simulink model "Position_Generator"  (R2017a)
settings: Solver=ode2  StartTime=0.0  StopTime=inf  FixedStep=0.001  RelTol=1e-3  EnableMultiTasking=on
model workspace (MAT data in the model file):
  Sig = Simulink.Signal
  Sig.DataType = 'auto'
  Sig.Dimensions = -1
  Sig.DimensionsMode = 'auto'
  Sig.Complexity = 'auto'
  Sig.SampleTime = -1
  Sig.SamplingMode = 'auto'
  video_step_size = 0.06
libraries: quarc_library x8, simulink x1
settings Model: SimulationMode=external  Creator=Admin  LastModifiedBy=mbohra
settings SolverCC: PositivePriorityOrder=on
settings OptimizationCC: LifeSpan=inf
settings DebuggingCC: ParameterPrecisionLossMsg=none  SFUnexpectedBacktrackingDiag=warning  SFNoUnconditionalDefaultTransitionDiag=warning  SFExecutionAtInitializationDiag=none
settings HardwareCC: ProdBitPerLong=64  ProdLargestAtomicFloat=None  ProdHWDeviceType=Intel->x86-64
settings RTWCC: SystemTargetFile=quarc_linux_x64.tlc  TemplateMakefile=quarc_linux_x64_tmf  Description=QUARC Linux x64 Target
settings STFCustomTargetCC: TargetLibSuffix=.a  TargetPreCompLibLocation=C:\PROGRA~3\QUARC\lib\2017a\LINUX_~1\release  ConcurrentExecutionCompliant=on  SystemTargetFile=quarc_linux_x64.tlc
settings GRTTargetCC: TargetLibSuffix=.a  TargetPreCompLibLocation=C:\PROGRA~3\QUARC\lib\2017a\LINUX_~1\release  TargetLangStandard=C89/C90 (ANSI)  ParMdlRefBuildCompliant=off  CompOptLevelCompliant=off  CombineOutputUpdateFcns=off  MatFileLogging=off  CPPClassGenCompliant=off  GRTInterface=on  UseToolchainInfoCompliant=off  ExtMode=on  ExtModeMexFile=quarc_comm  ExtModeMexArgs='-w -d /tmp -uri %u -IP_address tcpip://192.168.2.3:18666','tcpip://qondor888864.local:17002?retries=10'
settings ConfigComp: CovMetricSettings=dw  CovHtmlReporting=on  CovSaveCumulativeToWorkspaceVar=on  CovSaveSingleToWorkspaceVar=on  CovExternalEMLEnable=off

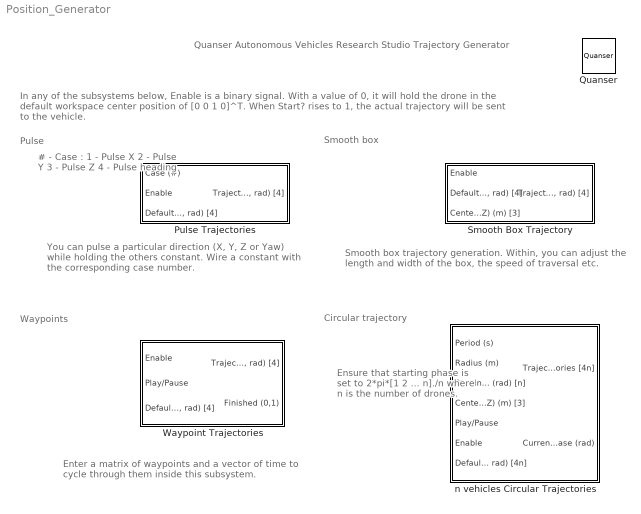
== system Position_Generator ==
  note: Ensure that starting phase is set to
      |  2*pi*[1 2 ... n]./n
      | where n is the number of drones.
  note: Circular trajectory
  note: Waypoints
  note: Smooth box
  note: Pulse
  note: You can pulse a particular direction (X, Y, Z or Yaw)
      | while holding the others constant. Wire a constant
      | with the corresponding case number.
  note: In any of the subsystems below, Enable is a binary signal. With a value of 0, it will hold the drone in the default workspace center position of [0 0 1 0]^T. When Start? rises to 1, the actual trajectory will be sent to the vehicle.
  note: # - Case :
      | 1 - Pulse X
      | 2 - Pulse Y
      | 3 - Pulse Z
      | 4 - Pulse heading
  note: Quanser Autonomous Vehicles Research Studio
      | Trajectory Generator
  note: Enter a matrix of waypoints and a vector of time
      | to cycle through them inside this subsystem.
  note: Smooth box trajectory generation. Within, you can adjust
      | the length and width of the box, the speed of traversal etc.
  Pulse Trajectories : Subsystem
  Quanser : quarc_library/Logos/Quanser
  Smooth Box Trajectory : Subsystem
  Waypoint Trajectories : Subsystem
  n vehicles Circular Trajectories : Subsystem

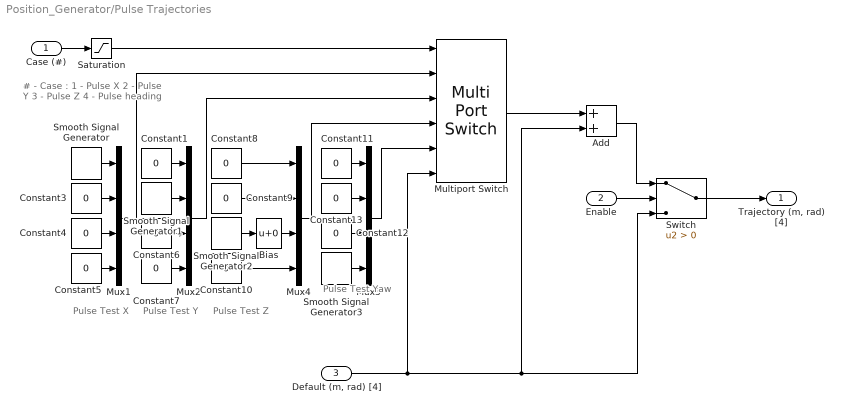
== system Position_Generator/Pulse Trajectories ==
  note: Pulse
      | Test Y
  note: Pulse
      | Test X
  note: Pulse
      | Test Z
  note: Pulse
      | Test
      | Yaw
  note: # - Case :
      | 1 - Pulse X
      | 2 - Pulse Y
      | 3 - Pulse Z
      | 4 - Pulse heading
  Case (#) : Inport
  Enable : Inport  Port=2
  "Default (m, rad) [4]" : Inport  Port=3
  Add : Sum
  Bias : Bias
  Constant{1,3..13} (12 alike) : Constant  Value=0
  Multiport Switch : MultiPortSwitch  Inputs=5
  Mux{1..2,4..5} (4 alike) : Mux  Inputs=[1 1 1 1]
  Saturation : Saturate  UpperLimit=5  LowerLimit=1
  Smooth Signal Generator : quarc_library/Sources/Signals/Smooth Signal Generator  signal_type=Square  source=Internal (dialog parameters)  amplitude=0.75  frequency=0.05  initial_phase=0  sample_time=qc_get_step_size  output_cos=off
      settings: SourceProductName=QUARC Targets
  Smooth Signal Generator1 : quarc_library/Sources/Signals/Smooth Signal Generator  signal_type=Square  source=Internal (dialog parameters)  amplitude=0.75  frequency=0.05  initial_phase=0  sample_time=qc_get_step_size  output_cos=off
      settings: SourceProductName=QUARC Targets
  Smooth Signal Generator2 : quarc_library/Sources/Signals/Smooth Signal Generator  signal_type=Square  source=Internal (dialog parameters)  amplitude=0.5  frequency=0.05  initial_phase=0  sample_time=qc_get_step_size  output_cos=off
      settings: SourceProductName=QUARC Targets
  Smooth Signal Generator3 : quarc_library/Sources/Signals/Smooth Signal Generator  signal_type=Square  source=Internal (dialog parameters)  amplitude=pi/4  frequency=0.05  initial_phase=0  sample_time=qc_get_step_size  output_cos=off
      settings: SourceProductName=QUARC Targets
  Switch : Switch  Criteria=u2 > Threshold
  "Trajectory (m, rad) [4]" : Outport
  wires:
  Constant3/1 -> Mux1/2
  Smooth Signal Generator/1 -> Mux1/1
  Constant5/1 -> Mux1/4
  Constant4/1 -> Mux1/3
  Mux1/1 -> Multiport Switch/2
  Case (#)/1 -> Saturation/1
  Mux2/1 -> Multiport Switch/3
  Constant6/1 -> Mux2/3
  Constant7/1 -> Mux2/4
  Constant1/1 -> Mux2/1
  Smooth Signal Generator1/1 -> Mux2/2
  Constant9/1 -> Mux4/2
  Constant8/1 -> Mux4/1
  Constant10/1 -> Mux4/4
  Smooth Signal Generator2/1 -> Bias/1
  Bias/1 -> Mux4/3
  Constant13/1 -> Mux5/2
  Constant11/1 -> Mux5/1
  Smooth Signal Generator3/1 -> Mux5/4
  Constant12/1 -> Mux5/3
  Mux4/1 -> Multiport Switch/4
  Mux5/1 -> Multiport Switch/5
  Saturation/1 -> Multiport Switch/1
  "Default (m, rad) [4]"/1 -> Add/2, Switch/3, Multiport Switch/6
  Switch/1 -> "Trajectory (m, rad) [4]"/1
  Enable/1 -> Switch/2
  Multiport Switch/1 -> Add/1
  Add/1 -> Switch/1

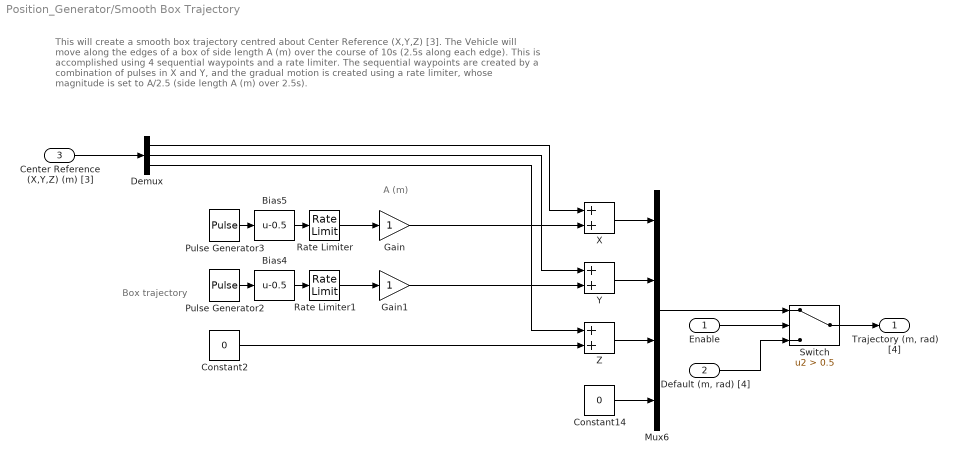
== system Position_Generator/Smooth Box Trajectory ==
  note: A (m)
  note: This will create a smooth box trajectory centred about Center Reference (X,Y,Z) [3]. The Vehicle will move along the edges of a box
      | of side length A (m) over the course of 10s (2.5s along each edge).
      |
      | This is accomplished using 4 sequential waypoints and a rate limiter. The sequential waypoints are created by a combination of
      | pulses in X and Y, and the gradual motion is created using a rate limiter, whose magnitude is set to A/2.5 (side length A (m) over 2.5s).
  note: Box
      | trajectory
  Enable : Inport
  "Default (m, rad) [4]" : Inport  Port=2
  Center Reference (X,Y,Z) (m) [3] : Inport  Port=3
  Bias4 : Bias  Bias=-0.5
  Bias5 : Bias  Bias=-0.5
  Constant14 : Constant  Value=0
  Constant2 : Constant  Value=0
  Demux : Demux  Outputs=3
  Gain : Gain
  Gain1 : Gain
  Mux6 : Mux  Inputs=[1 1 1 1]
  Pulse Generator2 : DiscretePulseGenerator  PulseType=Time based  Period=10  PulseWidth=50
  Pulse Generator3 : DiscretePulseGenerator  PulseType=Time based  Period=10  PulseWidth=50  PhaseDelay=-2.5
  Rate Limiter : RateLimiter  RisingSlewLimit=1/2.5  FallingSlewLimit=-1/2.5  SampleTimeMode=inherited  InitialCondition=0.5
  Rate Limiter1 : RateLimiter  RisingSlewLimit=1/2.5  FallingSlewLimit=-1/2.5  SampleTimeMode=inherited  InitialCondition=0.5
  Switch : Switch  Criteria=u2 > Threshold  Threshold=0.5
  X : Sum
  Y : Sum
  Z : Sum
  "Trajectory (m, rad) [4]" : Outport
  wires:
  Constant14/1 -> Mux6/4
  Bias5/1 -> Rate Limiter/1
  Pulse Generator3/1 -> Bias5/1
  Pulse Generator2/1 -> Bias4/1
  Bias4/1 -> Rate Limiter1/1
  Rate Limiter1/1 -> Gain1/1
  Rate Limiter/1 -> Gain/1
  "Default (m, rad) [4]"/1 -> Switch/3
  Switch/1 -> "Trajectory (m, rad) [4]"/1
  Enable/1 -> Switch/2
  Gain1/1 -> Y/2
  Demux/3 -> Z/1
  Center Reference (X,Y,Z) (m) [3]/1 -> Demux/1
  Demux/1 -> X/1
  Demux/2 -> Y/1
  Gain/1 -> X/2
  Constant2/1 -> Z/2
  X/1 -> Mux6/1
  Y/1 -> Mux6/2
  Z/1 -> Mux6/3
  Mux6/1 -> Switch/1

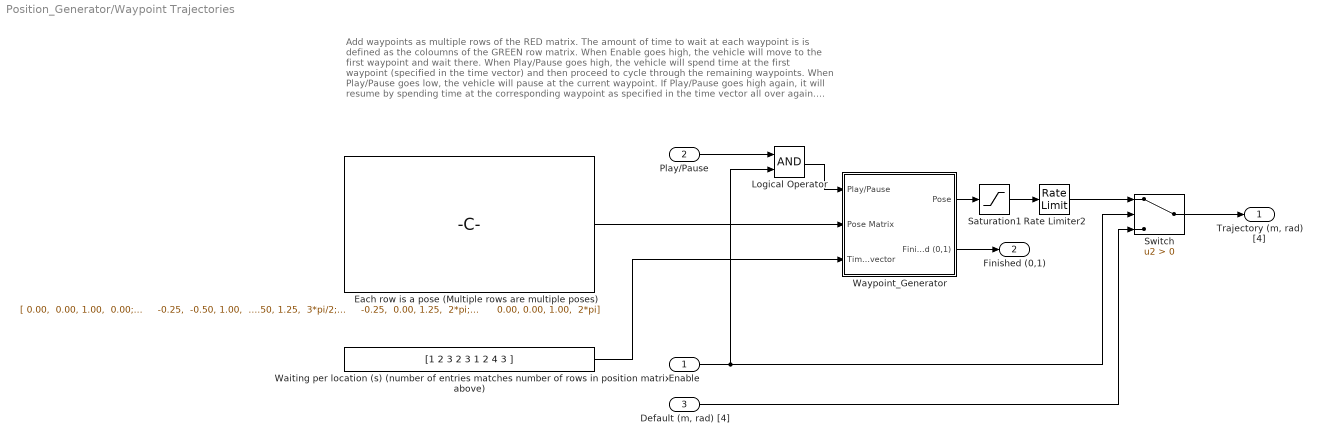
== system Position_Generator/Waypoint Trajectories ==
  note: Add waypoints as multiple rows of the RED matrix. The amount of time to wait at each waypoint is is defined as the coloumns of the GREEN row matrix.
      |
      | When Enable goes high, the vehicle will move to the first waypoint and wait there.
      | When Play/Pause goes high, the vehicle will spend time at the first waypoint (specified in the time vector) and then proceed to cycle through the remaining waypoints.
      | When Play/Pause goes low, the vehicle will pause at the current waypoint. If Play/Pause goes high again, it will resume by spending time at the corresponding waypoint
      | as specified in the time vector all over again.
      | When Enable goes low at any point, the vehicle will move back to the Default pose.
  Enable : Inport
  Play/Pause : Inport  Port=2
  "Default (m, rad) [4]" : Inport  Port=3
  Each row is a pose (Multiple rows are multiple poses) : Constant  Value=|
      | [ 0.00,  0.00, 1.00,  0.00;...
      |     -0.25,  -0.50, 1.00,  0.00;...
      |     -0.25, -0.50, 0.75,  0.00;...
      |      0.75, -0.50, 0.75,  pi/2;...
      |      0.75, -0.50, 1.25,  pi/2;...
      |      0.75,  0.50, 1.25,  pi;...
      |     -0.25,  0.50, 1.25,  3*pi/2;...
      |     -0.25,  0.00, 1.25,  2*pi;...
      |      0.00, 0.00, 1.00,  2*pi]
  Logical Operator : Logic  AllPortsSameDT=off  OutDataTypeStr=boolean
  Rate Limiter2 : RateLimiter  RisingSlewLimit=[1/3 1/3 1/6 pi/6]  FallingSlewLimit=[-1/3 -1/3 -1/6 -pi/6]  SampleTimeMode=inherited
  Saturation1 : Saturate  UpperLimit=[1.5 1.5 2 3*pi]  LowerLimit=[-1.5 -1.5 0 -3*pi]
  Switch : Switch  Criteria=u2 > Threshold
  Waiting per location (s) (number of entries matches number of rows in position matrix above) : Constant  Value=[1 2 3 2 3 1 2 4 3 ]
  Waypoint_Generator : Subsystem
  "Trajectory (m, rad) [4]" : Outport
  Finished (0,1) : Outport  Port=2
  wires:
  Waypoint_Generator/1(Pose) -> Saturation1/1
  Waiting per location (s) (number of entries matches number of rows in position matrix above)/1 -> Waypoint_Generator/3(Time vector)
  Each row is a pose (Multiple rows are multiple poses)/1 -> Waypoint_Generator/2(Pose Matrix)
  Saturation1/1 -> Rate Limiter2/1
  Play/Pause/1 -> Logical Operator/1
  Rate Limiter2/1 -> Switch/1
  Enable/1 -> Logical Operator/2, Switch/2
  "Default (m, rad) [4]"/1 -> Switch/3
  Switch/1 -> "Trajectory (m, rad) [4]"/1
  Logical Operator/1 -> Waypoint_Generator/1(Play/Pause)
  Waypoint_Generator/2(Finished (0,1)) -> Finished (0,1)/1

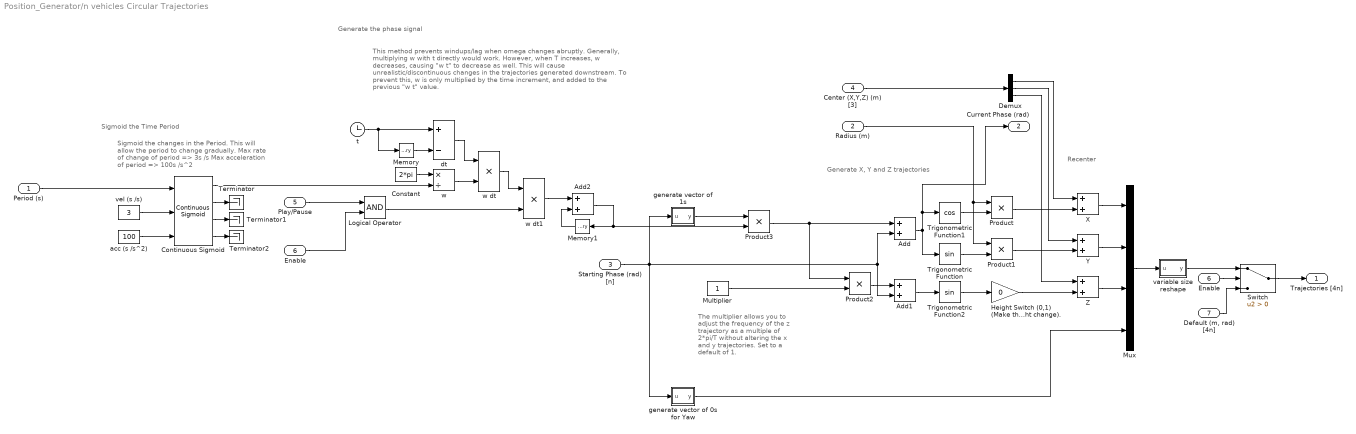
== system Position_Generator/n vehicles Circular Trajectories ==
  note: Recenter
  note: Generate X, Y and Z trajectories
  note: Generate the phase signal
  note: Sigmoid the changes in the Period. This will
      | allow the period to change gradually.
      | Max rate of change of period => 3s /s
      | Max acceleration of period => 100s /s^2
  note: Sigmoid the Time Period
  note: The multiplier allows you to adjust the frequency of the z trajectory as a multiple of 2*pi/T without altering the x and y trajectories. Set to a default of 1.
  note: This method prevents windups/lag when omega changes abruptly. Generally, multiplying w with t directly would work. However, when T increases, w decreases, causing "w t" to decrease as well. This will cause unrealistic/discontinuous changes in the trajectories generated downstream.
      |
      | To prevent this, w is only multiplied by the time increment, and added to the previous "w t" value.
  Period (s) : Inport
  Radius (m) : Inport  Port=2
  Starting Phase (rad) [n] : Inport  Port=3
  Center (X,Y,Z) (m) [3] : Inport  Port=4
  Play/Pause : Inport  Port=5
  Enable : Inport  Port=6
  "Default (m, rad) [4n]" : Inport  Port=7
  " Enable " : InportShadow  Port=6
  Add : Sum
  Add1 : Sum
  Add2 : Sum
  Constant : Constant  Value=2*pi
  Continuous Sigmoid : quarc_library/Sources/Sigmoids/Continuous Sigmoid  params_source=External (input ports)  max_velocity=2  max_acceleration=10  initial_position=10  initial_velocity=0  hold_off=0.5  input_sample_time=-1  output_sample_time=qc_get_step_size
      settings: SourceProductName=QUARC Targets
  Demux : Demux  Outputs=3
  Height Switch (0,1) (Make this 0 to disable height change). : Gain  Gain=0
  Logical Operator : Logic  AllPortsSameDT=off  OutDataTypeStr=boolean
  Memory : Memory
  Memory1 : Memory
  Multiplier : Constant
  Mux : Mux
  Product{,1..3} (4 alike) : Product
  Switch : Switch  Criteria=u2 > Threshold
  Terminator : Terminator
  Terminator1 : Terminator
  Terminator2 : Terminator
  Trigonometric Function : Trigonometry
  Trigonometric Function1 : Trigonometry  Operator=cos
  Trigonometric Function2 : Trigonometry
  X : Sum
  Y : Sum
  Z : Sum
  acc (s /s^2) : Constant  Value=100
  dt : Sum  Inputs=+-
  generate vector of 0s for Yaw : MATLAB Function  TreatAsAtomicUnit=on
  generate vector of 1s : MATLAB Function  TreatAsAtomicUnit=on
  t : Clock
  variable size reshape : MATLAB Function  TreatAsAtomicUnit=on
  vel (s /s) : Constant  Value=3
  w : Product  Inputs=*/
  w dt : Product
  w dt1 : Product
  Trajectories [4n] : Outport
  Current Phase (rad) : Outport  Port=2
  wires:
  Trigonometric Function/1 -> Product1/2
  Trigonometric Function1/1 -> Product/2
  Height Switch (0,1) (Make this 0 to disable height change)./1 -> Z/2
  Product1/1 -> Y/2
  Product/1 -> X/2
  Radius (m)/1 -> Product/1, Product1/1
  generate vector of 0s for Yaw/1(y) -> Mux/4
  Continuous Sigmoid/4 -> Terminator2/1
  Period (s)/1 -> Continuous Sigmoid/1
  Continuous Sigmoid/2 -> Terminator/1
  Continuous Sigmoid/3 -> Terminator1/1
  acc (s /s^2)/1 -> Continuous Sigmoid/3
  vel (s /s)/1 -> Continuous Sigmoid/2
  Add1/1 -> Trigonometric Function2/1
  Multiplier/1 -> Product2/2
  Product2/1 -> Add1/1
  Starting Phase (rad) [n]/1 -> Add/2, Add1/2, generate vector of 1s/1(u), generate vector of 0s for Yaw/1(u)
  Add2/1 -> Memory1/1, Product3/2
  Add/1 -> Current Phase (rad)/1, Trigonometric Function1/1, Trigonometric Function/1
  Center (X,Y,Z) (m) [3]/1 -> Demux/1
  Demux/2 -> Y/1
  Demux/1 -> X/1
  Trigonometric Function2/1 -> Height Switch (0,1) (Make this 0 to disable height change)./1
  Demux/3 -> Z/1
  X/1 -> Mux/1
  Y/1 -> Mux/2
  Z/1 -> Mux/3
  Memory/1 -> dt/2
  w dt/1 -> w dt1/1
  w dt1/1 -> Add2/1
  Constant/1 -> w/1
  Memory1/1 -> Add2/2
  w/1 -> w dt/2
  Continuous Sigmoid/1 -> w/2
  t/1 -> Memory/1, dt/1
  dt/1 -> w dt/1
  Mux/1 -> variable size reshape/1(u)
  Switch/1 -> Trajectories [4n]/1
  "Default (m, rad) [4n]"/1 -> Switch/3
  Enable/1 -> Switch/2
  Play/Pause/1 -> Logical Operator/1
  " Enable "/1 -> Logical Operator/2
  Logical Operator/1 -> w dt1/2
  Product3/1 -> Add/1, Product2/1
  generate vector of 1s/1(y) -> Product3/1
  variable size reshape/1(y) -> Switch/1

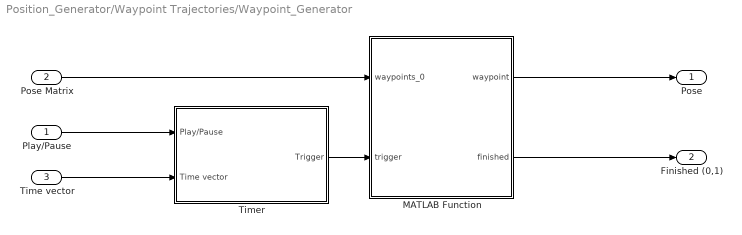
== system Position_Generator/Waypoint Trajectories/Waypoint_Generator ==
  Play/Pause : Inport
  Pose Matrix : Inport  Port=2
  Time vector : Inport  Port=3
  MATLAB Function : MATLAB Function  TreatAsAtomicUnit=on
  Timer : Subsystem
  Pose : Outport
  Finished (0,1) : Outport  Port=2
  wires:
  Pose Matrix/1 -> MATLAB Function/1(waypoints_0)
  MATLAB Function/1(waypoint) -> Pose/1
  Play/Pause/1 -> Timer/1(Play/Pause)
  Time vector/1 -> Timer/2(Time vector)
  Timer/1(Trigger) -> MATLAB Function/2(trigger)
  MATLAB Function/2(finished) -> Finished (0,1)/1

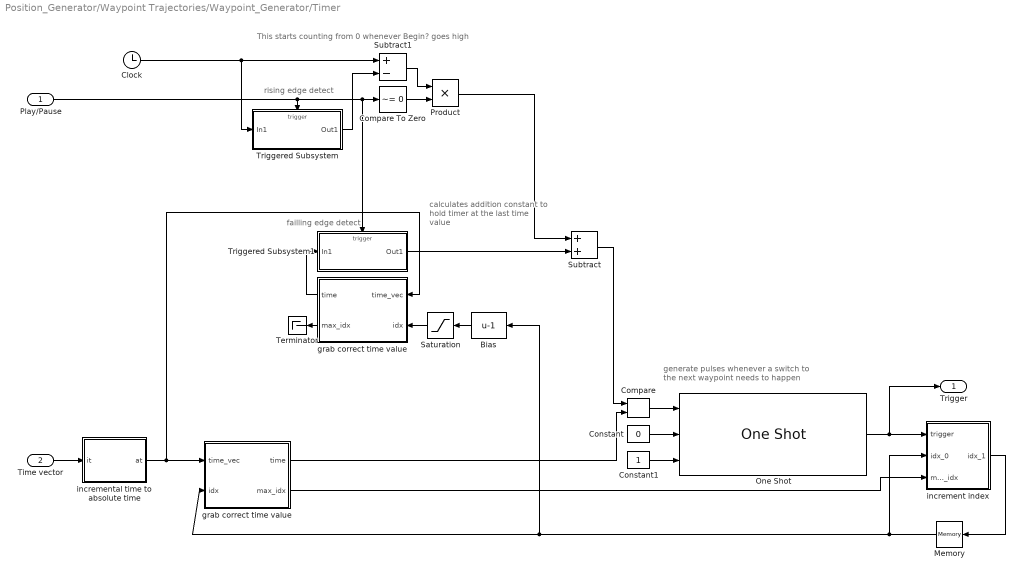
== system Position_Generator/Waypoint Trajectories/Waypoint_Generator/Timer ==
  note: generate pulses whenever a switch to
      |  the next waypoint needs to happen
  note: calculates addition constant to hold timer
      | at the last time value
  note: failling edge detect
  note: rising edge detect
  note: This starts counting from 0 whenever Begin? goes high
  Play/Pause : Inport
  Time vector : Inport  Port=2
  " grab correct time value " : MATLAB Function  TreatAsAtomicUnit=on
  Bias : Bias  Bias=-1
  Clock : Clock
  Compare : quarc_library/Logic Operations/Compare  operator=>=  output_data_type=boolean
      settings: SourceProductName=QUARC Targets
  Compare To Zero : simulink/Logic and Bit Operations/Compare To Zero  relop=~=  OutDataTypeStr=boolean
  Constant : Constant  Value=0
  Constant1 : Constant
  Memory : Memory  X0=1
  One Shot : quarc_library/Discontinuities/One Shot  trigger_type=Rising edge  redun_pulse=Ignore extraneous pulse  width_source=Specify via dialog  pulse_width=1
      settings: SourceProductName=QUARC Targets
  Product : Product
  Saturation : Saturate  UpperLimit=Inf  LowerLimit=1
  Subtract : Sum
  Subtract1 : Sum  Inputs=+-
  Terminator : Terminator
  Triggered Subsystem : Subsystem  TreatAsAtomicUnit=on
  Triggered Subsystem1 : Subsystem  TreatAsAtomicUnit=on
  grab correct time value : MATLAB Function  TreatAsAtomicUnit=on
  increment index : MATLAB Function  TreatAsAtomicUnit=on
  incremental time to absolute time : MATLAB Function  TreatAsAtomicUnit=on
  Trigger : Outport
  wires:
  Subtract1/1 -> Product/1
  Play/Pause/1 -> Triggered Subsystem/Trigger, Compare To Zero/1, Triggered Subsystem1/Trigger
  Triggered Subsystem/1(Out1) -> Subtract1/2
  Clock/1 -> Subtract1/1, Triggered Subsystem/1(In1)
  Compare To Zero/1 -> Product/2
  Subtract/1 -> Compare/1
  Time vector/1 -> incremental time to absolute time/1(it)
  increment index/1(idx_1) -> Memory/1
  grab correct time value/1(time) -> Compare/2
  Compare/1 -> One Shot/1
  Constant/1 -> One Shot/2
  Constant1/1 -> One Shot/3
  One Shot/1 -> increment index/1(trigger), Trigger/1
  Memory/1 -> Bias/1, grab correct time value/2(idx), increment index/2(idx_0)
  grab correct time value/2(max_idx) -> increment index/3(max_idx)
  Triggered Subsystem1/1(Out1) -> Subtract/2
  Product/1 -> Subtract/1
  Bias/1 -> Saturation/1
  incremental time to absolute time/1(at) -> " grab correct time value "/1(time_vec), grab correct time value/1(time_vec)
  " grab correct time value "/2(max_idx) -> Terminator/1
  " grab correct time value "/1(time) -> Triggered Subsystem1/1(In1)
  Saturation/1 -> " grab correct time value "/2(idx)

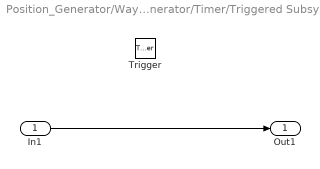
== system Position_Generator/Waypoint Trajectories/Waypoint_Generator/Timer/Triggered Subsystem ==
  In1 : Inport
  Trigger : TriggerPort  VariantControl=Variant
  Out1 : Outport
  wires:
  In1/1 -> Out1/1

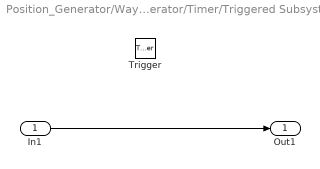
== system Position_Generator/Waypoint Trajectories/Waypoint_Generator/Timer/Triggered Subsystem1 ==
  In1 : Inport
  Trigger : TriggerPort  TriggerType=falling  VariantControl=Variant
  Out1 : Outport
  wires:
  In1/1 -> Out1/1

== matlab function Position_Generator/n vehicles Circular Trajectories/generate vector of 0s for Yaw ==
  data: u input; y output
function y = fcn(u)

y = 0.*u;

== matlab function Position_Generator/n vehicles Circular Trajectories/generate vector of 1s ==
  data: u input; y output
function y = fcn(u)

y = 0.*u + 1;

== matlab function Position_Generator/Waypoint Trajectories/Waypoint_Generator/MATLAB Function ==
  data: waypoints_0 input; waypoint output; trigger input; finished output
function [waypoint, finished]  = fcn(waypoints_0, trigger)
persistent idx;
[m, ~] = size(waypoints_0);
finished = 0;
if isempty(idx)
    idx = 1;
end

if trigger && idx < m
    idx = idx + 1;
end

if idx == m
    finished = 1;
end

waypoint = waypoints_0(idx, :);

== matlab function Position_Generator/Waypoint Trajectories/Waypoint_Generator/Timer/ grab correct time value  ==
  data: time_vec input; time output; idx input; max_idx output
function [time, max_idx] = fcn(time_vec, idx)

time = time_vec(idx);
max_idx = length(time_vec);

== matlab function Position_Generator/Waypoint Trajectories/Waypoint_Generator/Timer/grab correct time value ==
  data: time_vec input; time output; idx input; max_idx output
function [time, max_idx] = fcn(time_vec, idx)

time = time_vec(idx);
max_idx = length(time_vec);

== matlab function Position_Generator/Waypoint Trajectories/Waypoint_Generator/Timer/increment index ==
  data: trigger input; idx_1 output; idx_0 input; max_idx input
function idx_1 = fcn(trigger, idx_0, max_idx)

if trigger && (idx_0 < max_idx)
    idx_1 = idx_0 + 1;
else
    idx_1 = idx_0;
end

== matlab function Position_Generator/Waypoint Trajectories/Waypoint_Generator/Timer/incremental time to absolute time ==
  data: it input; at output
function at = fcn(it)
at = it;
n = length(it);
for i = 2:n
    at(i) = at(i-1) + it(i); 
end

== matlab function Position_Generator/n vehicles Circular Trajectories/variable size reshape ==
  data: u input; y output
function y = fcn(u)
y = u;
num = length(u)/4;
for i = 1:4
    for j = 1:num
        y(4*(j-1) + i) = u(j + num*(i-1));
    end
end
